simulink model "WLV"  (R2022b)
settings: Solver=VariableStepAuto  StartTime=0  StopTime=18  RelTol=1e-3  AbsTol=1e-3
values from neighbouring files (symbols this model uses):
  s = t / T    [vx.m]
undefined symbols (not defined in the file or in its folder): X, Y, Z
libraries: sm_lib x108, nesl_utility x44, slpidlib x9
(part 4 of 4)

== system WLV/Subsystem/髋RR ==
  Rigid Transform17 : sm_lib/Frames and Transforms/Rigid Transform  TranslationMethod=StandardAxis  TranslationStandardOffset=-0.03/2  TranslationLengthUnit=m  TranslationStandardAxis=+Y  TranslationCartesianOffset=[0.15 0.01 0]  TranslationROffset=0  TranslationROffsetUnits=m  TranslationZOffset=0  TranslationZOffsetUnits=m  TranslationThetaOffset=0  TranslationThetaOffsetUnits=deg  RotationMethod=StandardAxis  RotationAngleUnits=deg  RotationStandardAxis=+X  RotationAngle=-90  RotationArbitraryAxis=[0 0 1]  FollAlignAxisA=+X  BaseAlignAxisA=+Y  FollAlignAxisB=+Y  BaseAlignAxisB=+Z  RotationSequenceAxes=FollowerAxes  RotationSequence=XYX  RotationSequenceAngles=[0 0 0]  RotationSequenceAnglesUnits=deg  RotationMatrix=[1 0 0; 0 1 0; 0 0 1]  Quaternion=[1 0 0 0]
  Rigid Transform29 : sm_lib/Frames and Transforms/Rigid Transform  TranslationMethod=StandardAxis  TranslationStandardOffset=-0.35/2  TranslationLengthUnit=m  TranslationStandardAxis=+Y  TranslationCartesianOffset=[0 0 0]  TranslationROffset=0  TranslationROffsetUnits=m  TranslationZOffset=0  TranslationZOffsetUnits=m  TranslationThetaOffset=0  TranslationThetaOffsetUnits=deg  RotationMethod=None  RotationAngleUnits=deg  RotationStandardAxis=+Z  RotationAngle=0.0  RotationArbitraryAxis=[0 0 1]  FollAlignAxisA=+X  BaseAlignAxisA=+Y  FollAlignAxisB=+Y  BaseAlignAxisB=+Z  RotationSequenceAxes=FollowerAxes  RotationSequence=XYX  RotationSequenceAngles=[0 0 0]  RotationSequenceAnglesUnits=deg  RotationMatrix=[1 0 0; 0 1 0; 0 0 1]  Quaternion=[1 0 0 0]
  髋电机_RR : sm_lib/Body Elements/Cylindrical Solid  GraphicAmbientColor=[0.15 0.15 0.15 1.0]  BasedOnType=Density  CenterOfMass=[0 0 0]  CenterOfMassUnits=m  GraphicDiffuseColor=[0.2 0.2 0.2]  CylinderLength=0.03  CylinderLengthUnits=m  CylinderRadius=0.03  CylinderRadiusUnits=m  Density=100  DensityUnits=kg/m^3  DoExposeReferenceFrame=off  GraphicEmissiveColor=[0.0 0.0 0.0 1.0]  ExportEntireGeometry=off  SerializedFrames=<Frames><Frame><Id>Frame1</Id><Value><Name>T</Name><Origin><Source>GeometricFeature</Source><FeatureName>top surface</FeatureName></Origin><PrimaryAxis><DefinedDirection>+Y</DefinedDirection><Source>ReferenceFrame</Source><SourceDirection>+Z</SourceDirection><FeatureName></FeatureName></PrimaryAxis><SecondaryAxis><DefinedDirection>+X</DefinedDirection><Source>ReferenceFrame</Source><SourceDirection>+X</SourceDirection><FeatureName></FeatureName></SecondaryAxis></Value></Frame></Frames>  MarkerShape=Sphere  MarkerSize=10  GraphicType=FromGeometry  InertiaType=CalculateFromGeometry  Mass=1  MassUnits=kg  MomentsOfInertia=[1 1 1]  MomentsOfInertiaUnits=kg*m^2  GraphicOpacity=1.0  ProductsOfInertia=[0 0 0]  ProductsOfInertiaUnits=kg*m^2  GraphicShininess=75  GraphicSpecularColor=[0.5 0.5 0.5 1.0]  GraphicVisPropType=SimpleVisualProperties
  Conn1 : PMIOPort  Side=Left
  Conn2 : PMIOPort  Port=2  Side=Right
  connections:
  髋电机_RR/LConn1 -- Rigid Transform29/RConn1 -- Rigid Transform17/LConn1
  Rigid Transform17/RConn1 -- Conn2/RConn1
  Conn1/RConn1 -- Rigid Transform29/LConn1

== matlab function WLV/Subsystem6/MATLAB Function ==
  data: t input; vx output
function vx = vx(t)
    v_max = 0.7;  % 目标速度
    T = 1;        % 上升时间长度（秒）

    if t <= 0
        vx = 0;
    elseif t < T
        s = t / T;
        vx = v_max * (3*s^2 - 2*s^3);  
    else
        vx = v_max;
    end
end

== matlab function WLV/Subsystem5/MATLAB Function4 ==
  data: t input; vx output
function vx = vx(t)
    v_max = 0.7;  % 目标速度
    T = 1;        % 上升时间长度（秒）

    if t <= 0
        vx = 0;
    elseif t < T
        s = t / T;
        vx = v_max * (3*s^2 - 2*s^3);  
    else
        vx = v_max;
    end
end

== matlab function WLV/Subsystem5/MATLAB Function1 ==
  data: fd_all input; rb_all input; Torque_all output
function Torque_all = JointTorque( fd_all,rb_all)
% 输入：
%   rb_all : [8×1] 4条腿的 [rbx1; rbz1; ... rbx4; rbz4]
%   fd_all : [8×1] 4条腿的 [fdx1; fdz1; ... fdx4; fdz4]
% 输出：
%   Torque_all : [8×1] 雅克比矩阵映射到每个轮腿的大腿和小腿关节前馈力矩

    L1 = 0.30;
    L2 = 0.29;
    g  = 9.81;
    mw = 2.4;
    torque_max = 144;

    % 初始化
    Torque_all = zeros(8,1);

    for i = 1:4
        idx = (i-1)*2 + 1;
        
        rb = rb_all(idx:idx+1);

        % 反解关节角
        [qh, qk] = Forward_Kinematics(rb, i);

        fd_x = fd_all(idx);
        fd_z = fd_all(idx+1) - mw * g;

        % 雅可比矩阵
        J = [ -L1*sin(qh) - L2*sin(qh + qk),  -L2*sin(qh + qk);
               L1*cos(qh) + L2*cos(qh + qk),   L2*cos(qh + qk) ];

        % 力 → 力矩
        torque_leg = J' * [fd_x; fd_z];

        % 限幅
        torque_leg = max(min(torque_leg, torque_max), -torque_max);

        Torque_all(idx:idx+1) = torque_leg;
    end
end

== matlab function WLV/Subsystem5/MATLAB Function ==
  data: X0 input; Uk output; X_ref_single input; I_ext input; gama_all input; rb_all input
function Uk= MPC_Controller(X0, X_ref_single, I_ext, gama_all, rb_all)
    % MPC_Controller - 基于当前状态和目标状态计算最优地面反作用力
    % rb_all:  [8x1] 列向量 [rb1x; rb1z; rb2x; rb2z; rb3x; rb3z; rb4x; rb4z]
    % gama_all:[4x1] 列向量 [gama1; gama2; gama3; gama4]

    %% ---------- 系统参数 ----------
    mb=60+9.6; mh=3.5; mk=1.5; mw=2.4;
    Lb=0.850; Lw=0.350; Lh=0.200;
    L1=0.300; L2=0.290; r=0.100; 
    g = 9.81;

    %% ---------- 初始化姿态 ----------
    theta = gama_all(1);

    %% ---------- 拆解输入 ----------
    rb1 = rb_all(1:2);
    rb2 = rb_all(3:4);
    rb3 = rb_all(5:6);
    rb4 = rb_all(7:8);

    gama1 = gama_all(1);
    gama2 = gama_all(2);
    gama3 = gama_all(3);
    gama4 = gama_all(4);

    rw1 = rb1 - [0; 0.1];
    rw2 = rb2 - [0; 0.1];
    rw3 = rb3 - [0; 0.1];
    rw4 = rb4 - [0; 0.1];

    %% ---------- 矩阵定义 ----------
    O2 = zeros(2); I2 = eye(2);
    R_theta = [cos(theta) 0; 0 1];
    Cross = [0 -1; 1 0];
    Iyy = (1/12) * mb * (Lb^2 + Lh^2);

    Rg1 = [cos(gama1) sin(gama1); -sin(gama1) cos(gama1)];
    Rg2 = [cos(gama2) sin(gama2); -sin(gama2) cos(gama2)];
    Rg3 = [cos(gama3) sin(gama3); -sin(gama3) cos(gama3)];
    Rg4 = [cos(gama4) sin(gama4); -sin(gama4) cos(gama4)];

    %% ---------- 状态空间模型 ----------
    nx = 8; nu = 8; Np = 20; Nc = 20;
    dt  = 0.1;

    A = [O2 O2 R_theta' O2;
         O2 O2 O2       I2;
         O2 O2 O2       O2;
         O2 O2 O2       O2];

    H = zeros(nx, nu);
    H(6,:)   = [1/Iyy*(Cross*Rg1*rb1)', 1/Iyy*(Cross*Rg2*rb2)', ...
                1/Iyy*(Cross*Rg3*rb3)', 1/Iyy*(Cross*Rg4*rb4)'];
    H(7:8,:) = [I2*Rg1/mb, I2*Rg2/mb, I2*Rg3/mb, I2*Rg4/mb];

    Hw = zeros(nx, nu);
    Hw(6,:)   = [1/Iyy*(Cross*Rg1*rw1)', 1/Iyy*(Cross*Rg2*rw2)', ...
                 1/Iyy*(Cross*Rg3*rw3)', 1/Iyy*(Cross*Rg4*rw4)'];
    Hw(7:8,:) = [I2*Rg1/mb, I2*Rg2/mb, I2*Rg3/mb, I2*Rg4/mb];

    G = [0;0;0;0;0;0;0;-g];

    % 离散化
    Ad  = eye(nx) + dt * A;
    Hd  = dt * H;
    Hwd = dt * Hw;
    Gd  = dt * G;

    % 权重矩阵
    Q_single = diag([1, 1, 1, 20, 1, 1, 1, 0.5]); 
    R_single = 1e-4*eye(nu);
    Q = kron(eye(Np), Q_single);
    R = kron(eye(Nc), R_single);

    % 目标轨迹序列
    X_ref = repmat(X_ref_single, Np, 1);

    %% ---------- 预测矩阵构建 ----------
    A_qp = zeros(nx*Np, nx);
    H_qp = zeros(nx*Np, nu*Nc);
    D_qp = zeros(nx*Np,1);
    for i = 1:Np
        A_qp((i-1)*nx+1:i*nx, :) = Ad^i;
        for j = 1:min(i,Nc)
            H_qp((i-1)*nx+1:i*nx, (j-1)*nu+1:j*nu) = Ad^(i-j)*Hd;
        end
        tempD = zeros(nx,1);
        for j = 0:i-1
            tempD = tempD + Ad^j * (Hwd * I_ext + Gd);
        end
        D_qp((i-1)*nx+1:i*nx) = tempD;
    end

    %% ---------- 构建QP问题 ----------
    H_qp_total = H_qp' * Q * H_qp + R;
    H_qp_total = 0.5 * (H_qp_total + H_qp_total');  % 强制对称
    f_qp = H_qp' * Q * (A_qp*X0 + D_qp - X_ref);

    coder.extrinsic('quadprog');
    U_opt = zeros(nu*Nc,1);
    U_opt = quadprog(H_qp_total, f_qp, [], [], [], [], [], [], [], []);
    Uk = U_opt(1:nu);
end

== matlab function WLV/Subsystem5/MATLAB Function2 ==
  data: Zw_all input; pdz output
function pdz = pdz(Zw_all)
% 输入:
%   Zw_all : [4x1] 当前轮子的 rbz
% 输出:
%   pdz    : 期望质心位置

    z_min = min(Zw_all);

    pdz = 0.28 + z_min;
end

== matlab function WLV/Subsystem1/MATLAB Function ==
  data: rb input; qh output; qk output; legIndex input
function [qh, qk] = Forward_Kinematics(rb, legIndex)
% 输入
% legIndex ：轮腿编号
% rb = [rbx; rbz]，腿轮相对质心的位置向量
% 输出
% qh, qk ：髋关节和膝关节角度（单位：弧度）
    
    % 参数设置
    L  = 0.850 - 0.05 * 2;  % 车体总长减去边缘
    L1 = 0.300;  % 大腿长度
    L2 = 0.290;  % 小腿长度

    % 解析输入
    x = rb(1);
    z = rb(2);
    
    % 计算 dx
    if ismember(legIndex, [1, 2])  % 前腿
        dx = x - L/2;
    else                           % 后腿
        dx = -x - L/2;
    end
    dz = z;
    r = sqrt(dx^2 + dz^2);  % 髋到轮心的距离

    % 计算膝关节角度 qk
    cos_qk = (r^2 - L1^2 - L2^2) / (2 * L1 * L2);
    cos_qk = max(min(cos_qk, 1), -1); 

    % 计算角度
    if ismember(legIndex, [1, 2])  % 前腿：膝关节向后弯
        qk = -acos(cos_qk);
        phi = atan2(-dz, dx);
        cos_psi = (L1^2 + r^2 - L2^2) / (2 * L1 * r);
        cos_psi = max(min(cos_psi, 1), -1);
        psi = acos(cos_psi);
        qh = phi + psi;
    else                           % 后腿：膝关节向前弯
        qk = acos(cos_qk);
        phi = atan2(-dz, dx);
        cos_psi = (L1^2 + r^2 - L2^2) / (2 * L1 * r);
        cos_psi = max(min(cos_psi, 1), -1);
        psi = acos(cos_psi);
        qh = pi - (phi + psi);
    end
end

== matlab function WLV/Subsystem2/MATLAB Function ==
  data: rb input; qh output; qk output; legIndex input
function [qh, qk] = Forward_Kinematics(rb, legIndex)
    % 输入: rb = [rbx; rbz]，腿轮相对质心的位置向量
    % 输出: qh, qk，髋关节和膝关节角度（单位：弧度）
    
    % 参数设置
    L  = 0.850 - 0.05 * 2;  % 车体总长减去边缘
    L1 = 0.300;  % 大腿长度
    L2 = 0.290;  % 小腿长度

    % 解析输入
    x = rb(1);
    z = rb(2);
    
    % 确保 legIndex 合法
    assert(ismember(legIndex, 1:4), 'Invalid legIndex');

    % 计算 dx
    if ismember(legIndex, [1, 2])  % 前腿
        dx = x - L/2;
    else                           % 后腿
        dx = -x - L/2;
    end
    dz = z;
    r = sqrt(dx^2 + dz^2);  % 髋到轮心的距离

    % 计算膝关节角度 qk，带数值保护
    cos_qk = (r^2 - L1^2 - L2^2) / (2 * L1 * L2);
    cos_qk = max(min(cos_qk, 1), -1);  % 避免超出 acos 定义域

    % 计算角度
    if ismember(legIndex, [1, 2])  % 前腿：膝关节向后弯
        qk = -acos(cos_qk);
        phi = atan2(-dz, dx);
        cos_psi = (L1^2 + r^2 - L2^2) / (2 * L1 * r);
        cos_psi = max(min(cos_psi, 1), -1);
        psi = acos(cos_psi);
        qh = phi + psi;
    else  % 后腿：膝关节向前弯
        qk = acos(cos_qk);
        phi = atan2(-dz, dx);
        cos_psi = (L1^2 + r^2 - L2^2) / (2 * L1 * r);
        cos_psi = max(min(cos_psi, 1), -1);
        psi = acos(cos_psi);
        qh = pi - (phi + psi);
    end
end

== matlab function WLV/Subsystem3/MATLAB Function ==
  data: rb input; qh output; qk output; legIndex input
function [qh, qk] = Forward_Kinematics(rb, legIndex)
    % 输入: rb = [rbx; rbz]，腿轮相对质心的位置向量
    % 输出: qh, qk，髋关节和膝关节角度（单位：弧度）
    
    % 参数设置
    L  = 0.850 - 0.05 * 2;  % 车体总长减去边缘
    L1 = 0.300;  % 大腿长度
    L2 = 0.290;  % 小腿长度

    % 解析输入
    x = rb(1);
    z = rb(2);
    
    % 确保 legIndex 合法
    assert(ismember(legIndex, 1:4), 'Invalid legIndex');

    % 计算 dx
    if ismember(legIndex, [1, 2])  % 前腿
        dx = x - L/2;
    else                           % 后腿
        dx = -x - L/2;
    end
    dz = z;
    r = sqrt(dx^2 + dz^2);  % 髋到轮心的距离

    % 计算膝关节角度 qk，带数值保护
    cos_qk = (r^2 - L1^2 - L2^2) / (2 * L1 * L2);
    cos_qk = max(min(cos_qk, 1), -1);  % 避免超出 acos 定义域

    % 计算角度
    if ismember(legIndex, [1, 2])  % 前腿：膝关节向后弯
        qk = -acos(cos_qk);
        phi = atan2(-dz, dx);
        cos_psi = (L1^2 + r^2 - L2^2) / (2 * L1 * r);
        cos_psi = max(min(cos_psi, 1), -1);
        psi = acos(cos_psi);
        qh = phi + psi;
    else  % 后腿：膝关节向前弯
        qk = acos(cos_qk);
        phi = atan2(-dz, dx);
        cos_psi = (L1^2 + r^2 - L2^2) / (2 * L1 * r);
        cos_psi = max(min(cos_psi, 1), -1);
        psi = acos(cos_psi);
        qh = pi - (phi + psi);
    end
end

== matlab function WLV/Subsystem4/MATLAB Function ==
  data: rb input; qh output; qk output; legIndex input
function [qh, qk] = Forward_Kinematics(rb, legIndex)
    % 输入: rb = [rbx; rbz]，腿轮相对质心的位置向量
    % 输出: qh, qk，髋关节和膝关节角度（单位：弧度）
    
    % 参数设置
    L  = 0.850 - 0.05 * 2;  % 车体总长减去边缘
    L1 = 0.300;  % 大腿长度
    L2 = 0.290;  % 小腿长度

    % 解析输入
    x = rb(1);
    z = rb(2);
    
    % 确保 legIndex 合法
    assert(ismember(legIndex, 1:4), 'Invalid legIndex');

    % 计算 dx
    if ismember(legIndex, [1, 2])  % 前腿
        dx = x - L/2;
    else                           % 后腿
        dx = -x - L/2;
    end
    dz = z;
    r = sqrt(dx^2 + dz^2);  % 髋到轮心的距离

    % 计算膝关节角度 qk，带数值保护
    cos_qk = (r^2 - L1^2 - L2^2) / (2 * L1 * L2);
    cos_qk = max(min(cos_qk, 1), -1);  % 避免超出 acos 定义域

    % 计算角度
    if ismember(legIndex, [1, 2])  % 前腿：膝关节向后弯
        qk = -acos(cos_qk);
        phi = atan2(-dz, dx);
        cos_psi = (L1^2 + r^2 - L2^2) / (2 * L1 * r);
        cos_psi = max(min(cos_psi, 1), -1);
        psi = acos(cos_psi);
        qh = phi + psi;
    else  % 后腿：膝关节向前弯
        qk = acos(cos_qk);
        phi = atan2(-dz, dx);
        cos_psi = (L1^2 + r^2 - L2^2) / (2 * L1 * r);
        cos_psi = max(min(cos_psi, 1), -1);
        psi = acos(cos_psi);
        qh = pi - (phi + psi);
    end
end

== matlab function WLV/MATLAB Function ==
  data: z input; rb_all output; gama_all input; Zw_all input
function rb_all = rb_now(z, gama_all, Zw_all)
% 输出 rb_all 为 8x1 向量
% 约束：rbz ∈ [-0.32, -0.17]

    qh = 146 * pi / 180;
    qk = -123 * pi / 180;
    L1 = 0.300;
    L2 = 0.290;
    L  = 0.850 - 0.05 * 2;

    % 初始化输出
    rb_all = zeros(8,1);

    % 横向坐标
    rbx_front =  L1*cos(qh) + L2*cos(qh + qk) + L/2;
    rbx_back  = -L1*cos(qh) - L2*cos(qh + qk) - L/2;

    for i = 1:4
        gamma = gama_all(i);
        Zw    = Zw_all(i);

        % 原始垂向距离
        rbz = ( - z + Zw) * cos(gamma);

        % 限制 rbz 在 [-0.32, -0.17]
        rbz = min(max(rbz, -0.32), -0.17);

        % 横向位置
        if i <= 2
            rbx = rbx_front;
        else
            rbx = rbx_back;
        end

        rb_all(2*i - 1) = rbx;
        rb_all(2*i    ) = rbz;
    end
end

== matlab function WLV/Subsystem5/MATLAB Function3 ==
  data: gama_all input; gama output
function gama = fcn(gama_all)
    gama = gama_all(1);
    
end

== matlab function WLV/Subsystem/Subsystem/MATLAB Function1 ==
  data: Zw_all input; z_max output; z_min output; delta_z output
function [z_max,z_min,delta_z] = pdz(Zw_all)
    z_min = min(Zw_all);
    z_max = max(Zw_all);
    delta_z = abs(z_max - z_min);
end

== matlab function WLV/Subsystem/Subsystem/MATLAB Function ==
  settings: updateMethod=DISCRETE
  data: xi input; zi input; gama_all output

function gama_all = GroundSlope(xi, zi)
% zi  : [4x1] 四个轮子的 z 轴高度
% xi  : [4x1] 四个轮子的 x 轴位置
% gamma : 估计地面倾角（rad）

    % 最小二乘拟合坡度
    x_mean = mean(xi);
    z_mean = mean(zi);
    
    numerator = sum((xi - x_mean) .* (zi - z_mean));
    denominator = sum((xi - x_mean).^2);
    
    a = numerator / denominator;
    gama = atan(a);  
    gama_all = [gama;gama;gama;gama]
end
